simulink model "TSCLAB_ModelPV_16"  (R2020a)
settings: Solver=VariableStepAuto  StartTime=0.0  StopTime=200  RelTol=1e-3
undefined symbols (not defined in the file or in its folder): serial
libraries: instrumentlib x3
settings Model: Creator=vasanza  LastModifiedBy=Familia Zúñiga Vega
settings DebuggingCC: ArithmeticOperatorsInVariantConditions=warning
settings SFSimCC: CustomCodeUndefinedFunction=UseInterfaceOnly

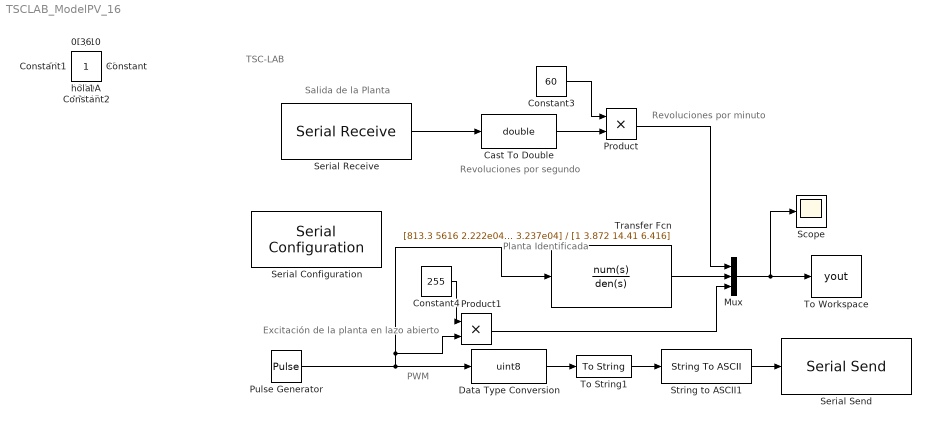
== system TSCLAB_ModelPV_16 ==
  note: PWM
  note: Excitación de la planta en lazo abierto
  note: Planta Identificada
  note: Revoluciones por minuto
  note: Revoluciones por segundo
  note: Salida de la Planta
  note: TSC-LAB
  Cast To Double : DataTypeConversion  OutDataTypeStr=double
  Constant3 : Constant  Value=60
  Constant4 : Constant  Value=255
  Data Type Conversion : DataTypeConversion  OutDataTypeStr=uint8
  Mux : Mux  Inputs=3
  Product : Product
  Product1 : Product
  Pulse Generator : DiscretePulseGenerator  PulseType=Time based  Period=26  PulseWidth=50
  Scope : Scope
  Serial Configuration : instrumentlib/Serial Configuration  Priority=-200000  ComPortMenu=COM7  ComPort=COM7  ObjConstructor=serial('COM7');  BaudRate=115200  DataBits=8  Parity=none  StopBits=1  FlowControl=none  Timeout=10  ByteOrder=LittleEndian
  Serial Receive : instrumentlib/Serial Receive  ComPortMenu=COM7  ComPort=COM7  ObjConstructor=serial('COM7');  Terminator=<none>  DataSize=[1 1]  DataType=uint8  EnableBlockingMode=on  ActionDataUnavailable=Output last received value  CustomValue=0  SampleTime=0.999
  Serial Send : instrumentlib/Serial Send  ComPortMenu=COM7  ComPort=COM7  ObjConstructor=serial('COM7');  Terminator=<none>  EnableBlockingMode=on
  String to ASCII1 : StringToASCII
  To String1 : ToString
  To Workspace : ToWorkspace  VariableName=yout  SampleTime=-1
      settings: Save2DSignal=2-D array (concatenate along first dimension)
  Transfer Fcn : TransferFcn  Numerator=[813.3 5616 2.222e04 3.237e04]  Denominator=[1 3.872 14.41 6.416]
  $ : Constant  IOType=siggen  Value=36
  , : Constant  IOType=siggen  Value=44
  {0,10,255,311,12345} (5 alike) : Constant  IOType=siggen
  0A : Constant  IOType=siggen  Value=10
  0D : Constant  IOType=siggen  Value=13
  13 : Constant  IOType=siggen  Value=13
  36 : Constant  IOType=siggen  Value=36
  Constant : Constant  IOType=siggen
  Constant1 : Constant  IOType=siggen
  Constant2 : Constant  IOType=siggen
  hola : Constant  IOType=siggen
  wires:
  Mux/1 -> Scope/1, To Workspace/1
  Data Type Conversion/1 -> To String1/1
  Serial Receive/1 -> Cast To Double/1
  Pulse Generator/1 -> Data Type Conversion/1, Product1/2, Transfer Fcn/1
  Cast To Double/1 -> Product/2
  Constant3/1 -> Product/1
  Product/1 -> Mux/1
  String to ASCII1/1 -> Serial Send/1
  To String1/1 -> String to ASCII1/1
  Transfer Fcn/1 -> Mux/2
  Constant4/1 -> Product1/1
  Product1/1 -> Mux/3
